simulink model "second_order_system_sim"  (R2023b)
settings: Solver=VariableStepAuto  StartTime=0.0  StopTime=10.0  RelTol=1e-3
settings Model: Creator=truel  LastModifiedBy=truel

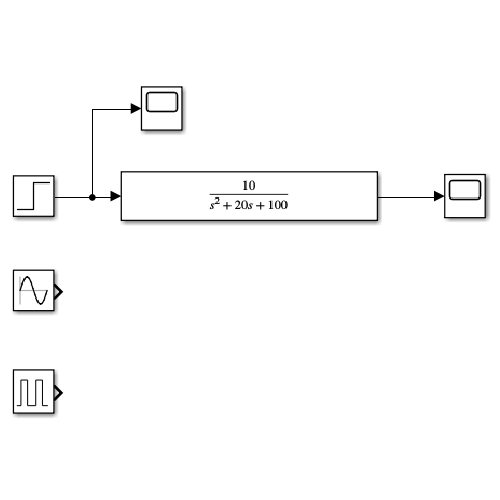
[thumbnail: Simulink's stored preview of the top-level diagram]
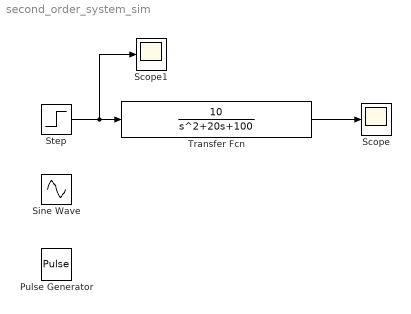
== system second_order_system_sim ==
  Pulse Generator : DiscretePulseGenerator  PulseType=Time based  Amplitude=1000  Period=0.001  PulseWidth=5
  Scope : Scope
  Scope1 : Scope
  Sine Wave : Sin  SampleTime=0
  Step : Step  SampleTime=0
  Transfer Fcn : TransferFcn  Numerator=[10]  Denominator=[1 20 100]
  wires:
  Transfer Fcn/1 -> Scope/1
  Step/1 -> Scope1/1, Transfer Fcn/1
